simulink model "ref_gen"  (Simulink 7.9)
settings: Solver=ode4  StartTime=0.0  StopTime=3  RelTol=1e-3
settings Model: Creator=James  LastModifiedBy=UW
settings DebuggingCC: FcnCallInpInsideContextMsg=Use local settings
settings GRTTargetCC: CombineOutputUpdateFcns=off  GRTInterface=on

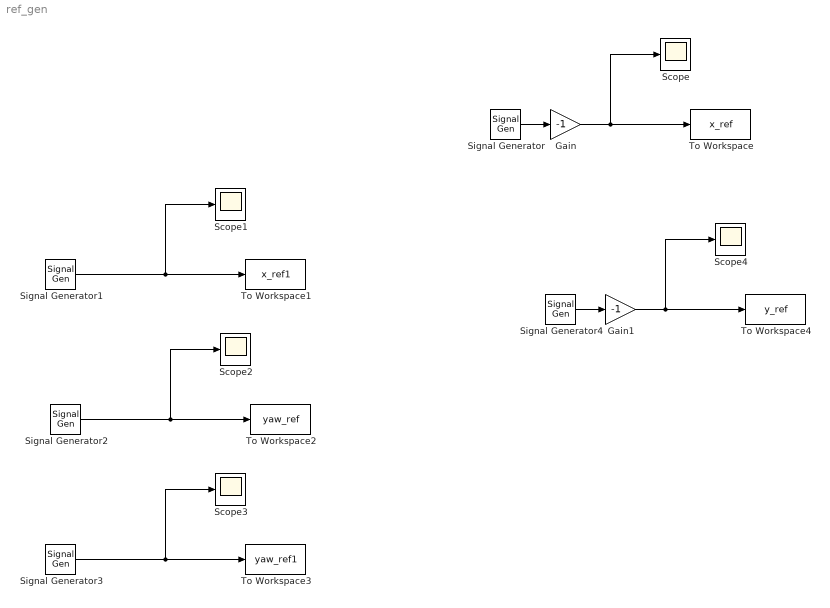
== system ref_gen ==
  Gain : Gain  Gain=-1
  Gain1 : Gain  Gain=-1
  Scope{,1..4} (5 alike) : Scope
      Scope settings: YMin=-600  YMax=600
      Scope1 settings: YMin=-600  YMax=600
      Scope2 settings: YMin=-600  YMax=600  SaveName=ScopeData2
      Scope3 settings: YMin=-600  YMax=600  SaveName=ScopeData3
      Scope4 settings: YMin=-600  YMax=600  SaveName=ScopeData4
  Signal Generator : SignalGenerator  WaveForm=square  Amplitude=300  Frequency=0.1
  Signal Generator1 : SignalGenerator  WaveForm=square  Amplitude=0  Frequency=0.0001
  Signal Generator2 : SignalGenerator  WaveForm=square  Amplitude=45  Frequency=0.0001
  Signal Generator3 : SignalGenerator  WaveForm=square  Amplitude=-45  Frequency=0.0001
  Signal Generator4 : SignalGenerator  WaveForm=square  Amplitude=1500  Frequency=0.1
  To Workspace : ToWorkspace  VariableName=x_ref  SampleTime=0.1
  To Workspace1 : ToWorkspace  VariableName=x_ref1  SampleTime=0.1
  To Workspace2 : ToWorkspace  VariableName=yaw_ref  SampleTime=0.1
  To Workspace3 : ToWorkspace  VariableName=yaw_ref1  SampleTime=0.1
  To Workspace4 : ToWorkspace  VariableName=y_ref  SampleTime=0.1
  wires:
  Signal Generator/1 -> Gain/1
  Signal Generator1/1 -> Scope1/1, To Workspace1/1
  Signal Generator2/1 -> To Workspace2/1, Scope2/1
  Gain/1 -> To Workspace/1, Scope/1
  Signal Generator3/1 -> Scope3/1, To Workspace3/1
  Signal Generator4/1 -> Gain1/1
  Gain1/1 -> Scope4/1, To Workspace4/1
